simulink model "Aerodynamic_coefficients"  (R2018a)
settings: Solver=VariableStepAuto  StartTime=0.0  StopTime=10.0  RelTol=1e-3
values from neighbouring files (symbols this model uses):
  CD0 = yD(find(~x))    [AOA_CL_CD_Cm.m]    (also in Linear_Coefficients.m = 0.051832)
  CDalpha = mean(diff(yD_linear)/d)    [AOA_CL_CD_Cm.m]    (also in Linear_Coefficients.m = 0.006587)
  CDdelta_e = 0.00036    [AOA_CL_CD_Cm.m]
  CL0 = yL(find(~x))    [AOA_CL_CD_Cm.m]    (also in Linear_Coefficients.m = 0.64791)
  CLalpha = mean(diff(yL_linear)/d)    [AOA_CL_CD_Cm.m]    (also in Linear_Coefficients.m = 0.088485)
  Clbeta = -0.00072    [AOA_CL_CD_Cm.m]    (also in Linear_Coefficients.m)
  Cldelta_a = -0.00393    [AOA_CL_CD_Cm.m]
  CLdelta_e = 0.00656    [AOA_CL_CD_Cm.m]    (also in Linear_Coefficients.m = 0.00328)
  Cldelta_r = -0.00008    (= -8e-05)    [AOA_CL_CD_Cm.m]
  Clp = -0.62    [AOA_CL_CD_Cm.m]    (also in Linear_Coefficients.m)
  Clr = -0.01    [AOA_CL_CD_Cm.m]    (also in Linear_Coefficients.m)
  Cm0 = ym(ZLI)    [AOA_CL_CD_Cm.m]    (also in Linear_Coefficients.m = -0.036061)
  Cmalpha = mean(diff(ym_linear)/d)    [AOA_CL_CD_Cm.m]    (also in Linear_Coefficients.m = -0.008902)
  Cmdelta_e = -0.01684    [AOA_CL_CD_Cm.m]    (also in Linear_Coefficients.m = -0.00842)
  Cnbeta = 0.00104    [AOA_CL_CD_Cm.m]    (also in Linear_Coefficients.m)
  Cndelta_a = 0.00034    [AOA_CL_CD_Cm.m]    (also in Linear_Coefficients.m)
  Cndelta_r = -0.00122    [AOA_CL_CD_Cm.m]    (also in Linear_Coefficients.m = -0.00061)
  Cnp = 0.004    [AOA_CL_CD_Cm.m]    (also in Linear_Coefficients.m)
  Cnr = -0.04    [AOA_CL_CD_Cm.m]    (also in Linear_Coefficients.m)
  CYbeta = -0.00668    [AOA_CL_CD_Cm.m]    (also in Linear_Coefficients.m)
  CYdelta_r = 0.00484    [AOA_CL_CD_Cm.m]    (also in Linear_Coefficients.m = 0.00242)
settings Model: Creator=McQueen_Zero  LastModifiedBy=McQueen_Zero

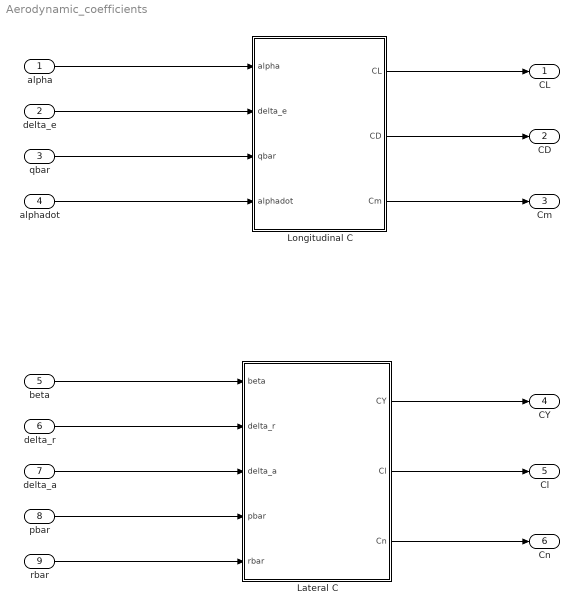
== system Aerodynamic_coefficients ==
  alpha : Inport
  delta_e : Inport  Port=2
  qbar : Inport  Port=3
  alphadot : Inport  Port=4
  beta : Inport  Port=5
  delta_r : Inport  Port=6
  delta_a : Inport  Port=7
  pbar : Inport  Port=8
  rbar : Inport  Port=9
  Lateral C : Subsystem
  Longitudinal C : Subsystem
  CL : Outport
  CD : Outport  Port=2
  Cm : Outport  Port=3
  CY : Outport  Port=4
  Cl : Outport  Port=5
  Cn : Outport  Port=6
  wires:
  alpha/1 -> Longitudinal C/1(alpha)
  delta_e/1 -> Longitudinal C/2(delta_e)
  qbar/1 -> Longitudinal C/3(qbar)
  alphadot/1 -> Longitudinal C/4(alphadot)
  Longitudinal C/1(CL) -> CL/1
  Longitudinal C/2(CD) -> CD/1
  Longitudinal C/3(Cm) -> Cm/1
  beta/1 -> Lateral C/1(beta)
  delta_r/1 -> Lateral C/2(delta_r)
  delta_a/1 -> Lateral C/3(delta_a)
  pbar/1 -> Lateral C/4(pbar)
  rbar/1 -> Lateral C/5(rbar)
  Lateral C/1(CY) -> CY/1
  Lateral C/2(Cl) -> Cl/1
  Lateral C/3(Cn) -> Cn/1

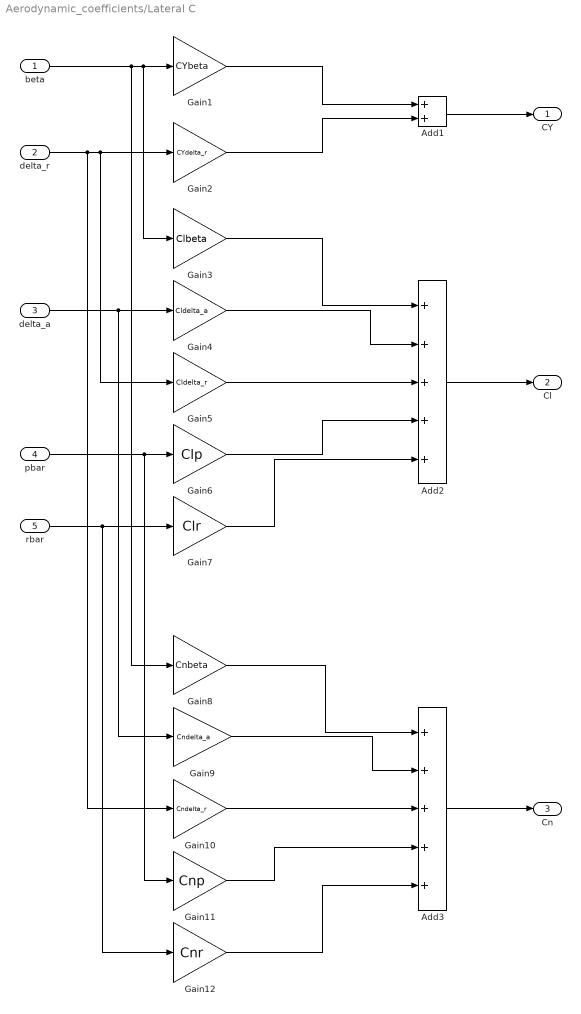
== system Aerodynamic_coefficients/Lateral C ==
  beta : Inport
  delta_r : Inport  Port=2
  delta_a : Inport  Port=3
  pbar : Inport  Port=4
  rbar : Inport  Port=5
  Add1 : Sum
  Add2 : Sum  Inputs=+++++
  Add3 : Sum  Inputs=+++++
  Gain1 : Gain  Gain=CYbeta
  Gain10 : Gain  Gain=Cndelta_r
  Gain11 : Gain  Gain=Cnp
  Gain12 : Gain  Gain=Cnr
  Gain2 : Gain  Gain=CYdelta_r
  Gain3 : Gain  Gain=Clbeta
  Gain4 : Gain  Gain=Cldelta_a
  Gain5 : Gain  Gain=Cldelta_r
  Gain6 : Gain  Gain=Clp
  Gain7 : Gain  Gain=Clr
  Gain8 : Gain  Gain=Cnbeta
  Gain9 : Gain  Gain=Cndelta_a
  CY : Outport
  Cl : Outport  Port=2
  Cn : Outport  Port=3
  wires:
  delta_r/1 -> Gain10/1, Gain5/1, Gain2/1
  beta/1 -> Gain8/1, Gain3/1, Gain1/1
  Gain12/1 -> Add3/5
  Add3/1 -> Cn/1
  pbar/1 -> Gain11/1, Gain6/1
  Gain1/1 -> Add1/1
  delta_a/1 -> Gain9/1, Gain4/1
  Gain2/1 -> Add1/2
  Gain5/1 -> Add2/3
  Gain11/1 -> Add3/4
  rbar/1 -> Gain12/1, Gain7/1
  Add2/1 -> Cl/1
  Gain9/1 -> Add3/2
  Gain4/1 -> Add2/2
  Gain3/1 -> Add2/1
  Add1/1 -> CY/1
  Gain8/1 -> Add3/1
  Gain6/1 -> Add2/4
  Gain10/1 -> Add3/3
  Gain7/1 -> Add2/5

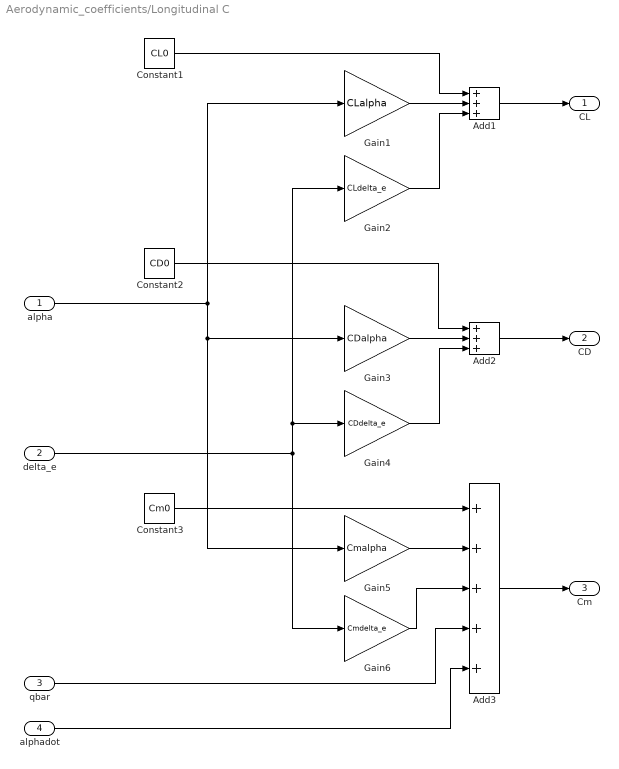
== system Aerodynamic_coefficients/Longitudinal C ==
  alpha : Inport
  delta_e : Inport  Port=2
  qbar : Inport  Port=3
  alphadot : Inport  Port=4
  Add1 : Sum  Inputs=+++
  Add2 : Sum  Inputs=+++
  Add3 : Sum  Inputs=+++++
  Constant1 : Constant  Value=CL0
  Constant2 : Constant  Value=CD0
  Constant3 : Constant  Value=Cm0
  Gain1 : Gain  Gain=CLalpha
  Gain2 : Gain  Gain=CLdelta_e
  Gain3 : Gain  Gain=CDalpha
  Gain4 : Gain  Gain=CDdelta_e
  Gain5 : Gain  Gain=Cmalpha
  Gain6 : Gain  Gain=Cmdelta_e
  CL : Outport
  CD : Outport  Port=2
  Cm : Outport  Port=3
  wires:
  Add1/1 -> CL/1
  Constant1/1 -> Add1/1
  Constant2/1 -> Add2/1
  Gain3/1 -> Add2/2
  Add2/1 -> CD/1
  Constant3/1 -> Add3/1
  Gain4/1 -> Add2/3
  alphadot/1 -> Add3/5
  Gain1/1 -> Add1/2
  Add3/1 -> Cm/1
  alpha/1 -> Gain3/1, Gain5/1, Gain1/1
  delta_e/1 -> Gain6/1, Gain4/1, Gain2/1
  Gain2/1 -> Add1/3
  Gain5/1 -> Add3/2
  Gain6/1 -> Add3/3
  qbar/1 -> Add3/4
